simulink model "DCPF_WithDroopNLload"  (R2015b)
settings: Solver=VariableStepAuto  StartTime=0.0  StopTime=1.0  RelTol=1e-3
undefined symbols (not defined in the file or in its folder): C_dc_link, V_dc_link_initial
libraries: powerlib x22
settings Model: Creator=Irina  LastModifiedBy=Irina

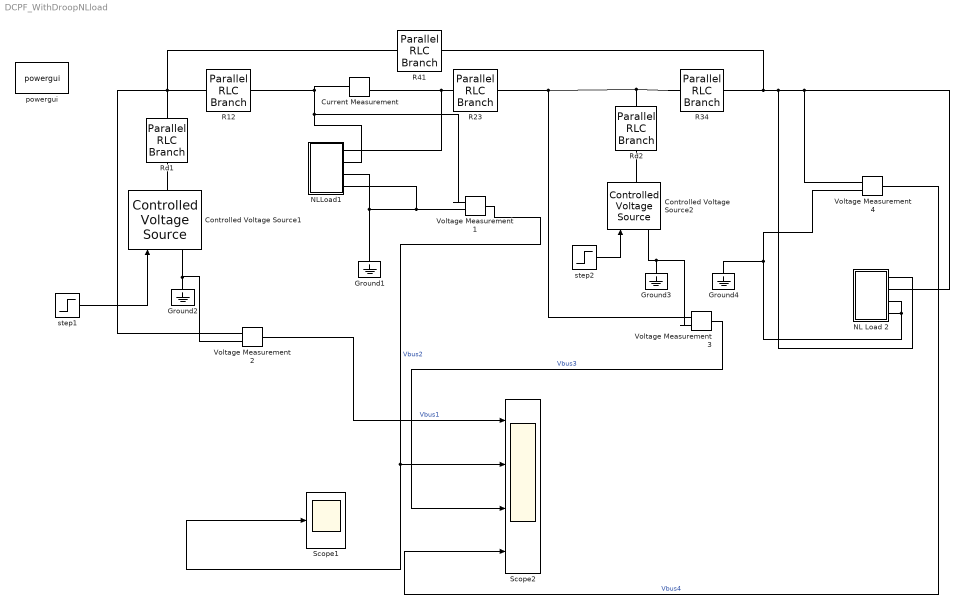
== system DCPF_WithDroopNLload ==
  Controlled Voltage Source1 : powerlib/Electrical Sources/Controlled Voltage Source  Initialize=on  Source_Type=DC  Amplitude=48  Phase=0  Frequency=0  Measurements=None
  Controlled Voltage Source2 : powerlib/Electrical Sources/Controlled Voltage Source  Initialize=on  Source_Type=DC  Amplitude=48  Phase=0  Frequency=0  Measurements=None
  Current Measurement : powerlib/Measurements/Current Measurement  PhasorSimulation=off  OutputType=Complex  PSBequivalent=0
  Ground{1..4} (4 alike) : powerlib/Elements/Ground  LConnTagsString=a
  NL Load 2 : Subsystem
  NLLoad1 : Subsystem
  R{12,23,34,41} (4 alike) : powerlib/Elements/Parallel RLC Branch  LConnTagsString=a  RConnTagsString=__new0  BranchType=R  Resistance=0.05  Inductance=1e-3  SetiL0=off  InitialCurrent=0  Capacitance=C_dc_link*2  Setx0=on  InitialVoltage=V_dc_link_initial/2  Measurements=None
  Rd1 : powerlib/Elements/Parallel RLC Branch  LConnTagsString=a  RConnTagsString=__new0  BranchType=R  Resistance=0.2  Inductance=1e-3  SetiL0=off  InitialCurrent=0  Capacitance=C_dc_link*2  Setx0=on  InitialVoltage=V_dc_link_initial/2  Measurements=None
  Rd2 : powerlib/Elements/Parallel RLC Branch  LConnTagsString=a  RConnTagsString=__new0  BranchType=R  Resistance=0.5  Inductance=1e-3  SetiL0=off  InitialCurrent=0  Capacitance=C_dc_link*2  Setx0=on  InitialVoltage=V_dc_link_initial/2  Measurements=None
  Scope1 : Scope
  Scope2 : Scope  NumInputPorts=4
  Voltage Measurement{1..4} (4 alike) : powerlib/Measurements/Voltage Measurement  PhasorSimulation=off  OutputType=Complex  PSBequivalent=0
  powergui : powerlib/powergui  Priority=1  SimulationMode=Continuous  SolverType=Tustin/Backward Euler (TBE)  SampleTime=50e-6  frequency=60  SPID=off  DisableSnubberDevices=off  DisableRonSwitches=off  DisableVfSwitches=off  SwTol=0  DisplayEquations=off  Interpol=off  ExternalGateDelay=off  methode=off  Ts=10  FunctionMessages=off  echomessages=off  HookPort=off  EnableUseOfTLC=off  x0status=blocks  frequencyindice=0  Pbase=100e6  ErrMax=1e-4  Iterations=50  UnitsV=kV  UnitsW=MW  buscounter=0  RestoreLinks=warning  ResistiveCurrentMeasurement=off  Frange=[0:2:500]  Ylog=off  Xlog=on  ShowGrid=off  save=off  variable=ZData  structure=0  ZoomFFT=off  StartTime=0.0  cycles=1  DisplayStyle=1  fundamental=60  FreqAxis=off  MaxFrequency=1000  frequencyindicesteady=1  RmsSteady=1  display=off
  step1 : Step  Time=0.01
  step2 : Step  Time=0.01
  wires:
  Voltage Measurement2/1 -> Scope2/1  "Vbus1"
  Voltage Measurement1/1 -> Scope1/1, Scope2/2  "Vbus2"
  Voltage Measurement3/1 -> Scope2/3  "Vbus3"
  Voltage Measurement4/1 -> Scope2/4  "Vbus4"
  step1/1 -> Controlled Voltage Source1/1
  step2/1 -> Controlled Voltage Source2/1
  connections:
  Rd1/LConn1 -- Controlled Voltage Source1/RConn1
  Rd1/RConn1 -- Voltage Measurement2/LConn1 -- R41/LConn1 -- R12/LConn1
  Ground3/LConn1 -- Controlled Voltage Source2/LConn1 -- Voltage Measurement3/LConn2
  Rd2/RConn1 -- R23/RConn1 -- Voltage Measurement3/LConn1 -- R34/LConn1
  Controlled Voltage Source2/RConn1 -- Rd2/LConn1
  Ground4/LConn1 -- Voltage Measurement4/LConn2 -- NL Load 2/RConn4 -- NL Load 2/RConn3
  R41/RConn1 -- NL Load 2/RConn1 -- Voltage Measurement4/LConn1 -- NL Load 2/RConn2 -- R34/RConn1
  Ground2/LConn1 -- Voltage Measurement2/LConn2 -- Controlled Voltage Source1/LConn1
  Current Measurement/RConn1 -- NLLoad1/RConn1 -- R23/LConn1
  Current Measurement/LConn1 -- NLLoad1/RConn2 -- Voltage Measurement1/LConn1 -- R12/RConn1
  Ground1/LConn1 -- NLLoad1/RConn3 -- NLLoad1/RConn4 -- Voltage Measurement1/LConn2

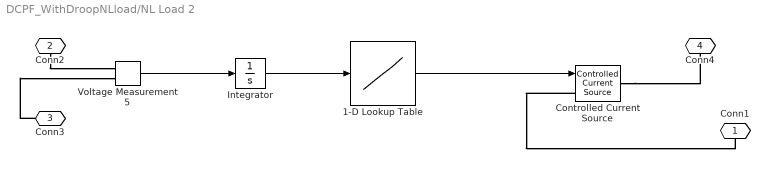
== system DCPF_WithDroopNLload/NL Load 2 ==
  1-D Lookup Table : Lookup_n-D  NumberOfTableDimensions=1  BreakpointsForDimension1=[-1.25 -1 1 1.25]*(230*sqrt(2)/(2*pi*50))  Table=[-2 -1 1 2]*(230*sqrt(2)/(4*pi*50))  InternalRulePriority=Speed  RndMeth=Simplest  InputSameDT=on
  Controlled Current Source : powerlib/Electrical Sources/Controlled Current Source  Initialize=on  Source_Type=AC  Amplitude=0  Phase=0  Frequency=0  Measurements=None
  Integrator : Integrator
  Voltage Measurement5 : powerlib/Measurements/Voltage Measurement  PhasorSimulation=off  OutputType=Complex  PSBequivalent=0
  Conn1 : PMIOPort  Port=1  Side=Right
  Conn2 : PMIOPort  Port=2  Side=Right
  Conn3 : PMIOPort  Port=3  Side=Right
  Conn4 : PMIOPort  Port=4  Side=Right
  wires:
  1-D Lookup Table/1 -> Controlled Current Source/1
  Voltage Measurement5/1 -> Integrator/1
  Integrator/1 -> 1-D Lookup Table/1
  connections:
  Conn3/RConn1 -- Voltage Measurement5/LConn2
  Controlled Current Source/RConn1 -- Conn4/RConn1
  Controlled Current Source/LConn1 -- Conn1/RConn1
  Conn2/RConn1 -- Voltage Measurement5/LConn1

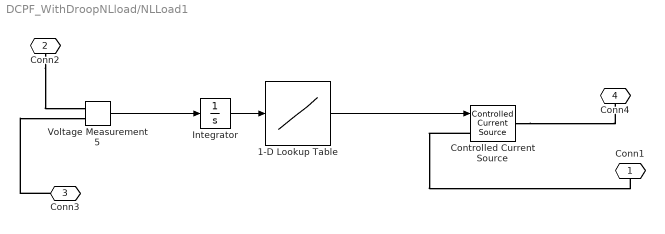
== system DCPF_WithDroopNLload/NLLoad1 ==
  1-D Lookup Table : Lookup_n-D  NumberOfTableDimensions=1  BreakpointsForDimension1=[-1.25 -1 1 1.25]*(230*sqrt(2)/(2*pi*50))  Table=[-2 -1 1 2]*(230*sqrt(2)/(4*pi*50))  InternalRulePriority=Speed  RndMeth=Simplest  InputSameDT=on
  Controlled Current Source : powerlib/Electrical Sources/Controlled Current Source  Initialize=on  Source_Type=AC  Amplitude=0  Phase=0  Frequency=0  Measurements=None
  Integrator : Integrator
  Voltage Measurement5 : powerlib/Measurements/Voltage Measurement  PhasorSimulation=off  OutputType=Complex  PSBequivalent=0
  Conn1 : PMIOPort  Port=1  Side=Right
  Conn2 : PMIOPort  Port=2  Side=Right
  Conn3 : PMIOPort  Port=3  Side=Right
  Conn4 : PMIOPort  Port=4  Side=Right
  wires:
  1-D Lookup Table/1 -> Controlled Current Source/1
  Voltage Measurement5/1 -> Integrator/1
  Integrator/1 -> 1-D Lookup Table/1
  connections:
  Conn3/RConn1 -- Voltage Measurement5/LConn2
  Controlled Current Source/RConn1 -- Conn4/RConn1
  Controlled Current Source/LConn1 -- Conn1/RConn1
  Conn2/RConn1 -- Voltage Measurement5/LConn1
